simulink model "single_track_ctrl_sim"  (R2020a)
settings: Solver=ode45  StartTime=0.0  StopTime=100  MaxStep=0.001  RelTol=1e-3
InitFcn:
  | single_ctrl_est_design
undefined symbols (not defined in the file): A, B, B1, C1, D1, K, kr
settings Model: Creator=jofr  LastModifiedBy=rizwanahmed
settings DataIOCC: LimitDataPoints=on  SaveFormat=Array  SignalLoggingSaveFormat=ModelDataLogs  ReturnWorkspaceOutputs=off
settings OptimizationCC: BlockReduction=off  BooleanDataType=off  LifeSpan=inf
settings DebuggingCC: SaveWithParameterizedLinksMsg=none  UnderspecifiedInitializationDetection=Classic  MergeDetectMultiDrivingBlocksExec=none  SignalResolutionControl=TryResolveAllWithWarning  MultiTaskDSMMsg=warning  MultiTaskCondExecSysMsg=none  SFUnexpectedBacktrackingDiag=warning  SFNoUnconditionalDefaultTransitionDiag=warning  SFExecutionAtInitializationDiag=none  ArithmeticOperatorsInVariantConditions=warning
settings HardwareCC: ProdBitPerPointer=32  ProdBitPerSizeT=32  ProdBitPerPtrDiffT=32  ProdLargestAtomicFloat=None  ProdIntDivRoundTo=Undefined  ProdEndianess=Unspecified  ProdWordSize=32  ProdHWDeviceType=32-bit Generic  TargetUnknown=on
settings ModelReferenceCC: PropagateSignalLabelsOutOfModel=off
settings SFSimCC: SimUseLocalCustomCode=off  CustomCodeUndefinedFunction=UseInterfaceOnly
settings RTWCC: RTWUseLocalCustomCode=off
settings CodeAppCC: StateflowObjectComments=on
settings GRTTargetCC: TargetLangStandard=C89/C90 (ANSI)
settings ConfigComp: CovMetricSettings=dw  CovHtmlReporting=on  CovSaveCumulativeToWorkspaceVar=on  CovSaveSingleToWorkspaceVar=on  CovExternalEMLEnable=off

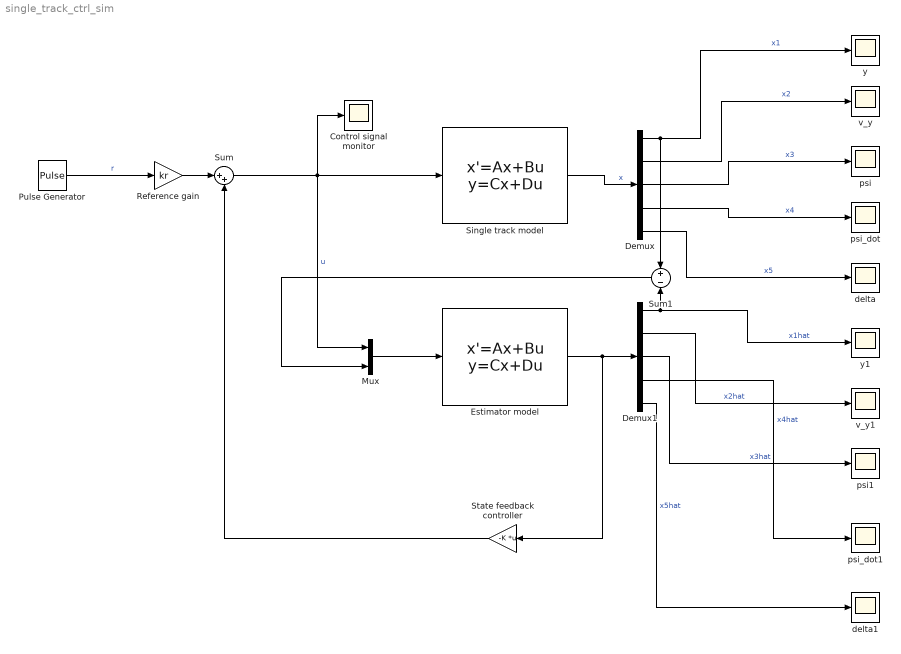
== system single_track_ctrl_sim ==
  Control signal monitor : Scope
  Demux : Demux  Outputs=5
  Demux1 : Demux  Outputs=5
  Estimator model : StateSpace  A=A  B=B1  C=C1  D=D1  InitialCondition=0
  Mux : Mux  Inputs=2
  Pulse Generator : DiscretePulseGenerator  PulseType=Time based  Amplitude=3.5  Period=40  PulseWidth=50  PhaseDelay=5
  Reference gain : Gain  Gain=kr
  Single track model : StateSpace  A=A  B=B  C=eye(5)  D=zeros(5,1)  InitialCondition=0
  State feedback controller : Gain  Gain=-K  Multiplication=Matrix(K*u)
  Sum : Sum  Inputs=|++
  Sum1 : Sum  Inputs=+|-
  delta : Scope
  delta1 : Scope
  psi : Scope
  psi1 : Scope
  psi_dot : Scope
  psi_dot1 : Scope
  v_y : Scope
  v_y1 : Scope
  y : Scope
  y1 : Scope
  wires:
  State feedback controller/1 -> Sum/2
  Demux1/4 -> psi_dot1/1  "x4hat"
  Reference gain/1 -> Sum/1
  Demux1/5 -> delta1/1  "x5hat"
  Demux/3 -> psi/1  "x3"
  Demux1/1 -> Sum1/2, y1/1  "x1hat"
  Estimator model/1 -> State feedback controller/1, Demux1/1
  Demux/4 -> psi_dot/1  "x4"
  Single track model/1 -> Demux/1  "x"
  Demux/1 -> Sum1/1, y/1  "x1"
  Sum1/1 -> Mux/2
  Demux1/3 -> psi1/1  "x3hat"
  Mux/1 -> Estimator model/1
  Demux/2 -> v_y/1  "x2"
  Sum/1 -> Mux/1, Single track model/1, Control signal monitor/1  "u"
  Pulse Generator/1 -> Reference gain/1  "r"
  Demux1/2 -> v_y1/1  "x2hat"
  Demux/5 -> delta/1  "x5"
